simulink model "CorN_TestBed"  (R2012b)
settings: Solver=FixedStepDiscrete  StartTime=0.0  StopTime=1  FixedStep=1  RelTol=1e-3
undefined symbols (not defined in the file): MWS
libraries: Lib_Cntrl_CorrectedSpeed_TMATS x1
settings Model: Creator=jwchapm2  LastModifiedBy=jwchapm2

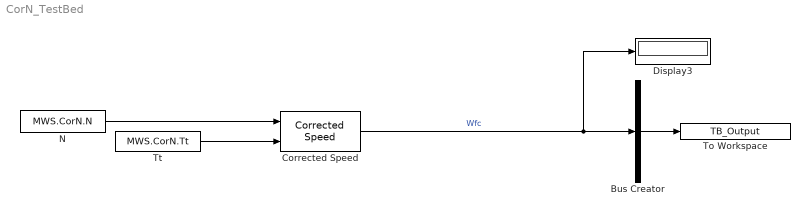
== system CorN_TestBed ==
  Bus Creator : BusCreator  Inputs=1
  Corrected Speed : Lib_Cntrl_CorrectedSpeed_TMATS/Corrected Speed  C_TSTD_M=MWS.CorN.TST
  Display3 : Display
  N : Constant  Value=MWS.CorN.N
  To Workspace : ToWorkspace  VariableName=TB_Output  SampleTime=-1
  Tt : Constant  Value=MWS.CorN.Tt
  wires:
  N/1 -> Corrected Speed/1
  Tt/1 -> Corrected Speed/2
  Corrected Speed/1 -> Bus Creator/1, Display3/1  "Wfc"
  Bus Creator/1 -> To Workspace/1
